simulink model "two_vector"  (R2018b)
settings: Solver=ode1  StartTime=0.0  StopTime=0.7  RelTol=1e-3
undefined symbols (not defined in the file): Ba, DiscIntNeverNeededParam, flux, Ki, Kp, L, R, states, Ts, v
libraries: powerlib x4, simulink x1
settings Model: SimulationMode=accelerator  Creator=123  LastModifiedBy=123
settings DebuggingCC: LibraryContextMissingDiagnostic=none
settings SFSimCC: SimUseLocalCustomCode=off
settings RTWCC: RTWUseLocalCustomCode=off

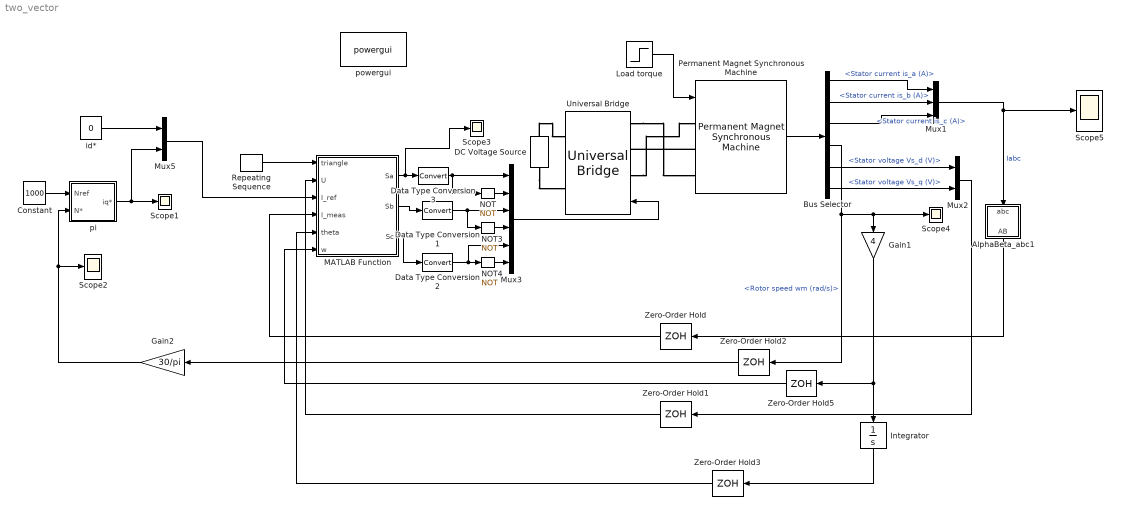
== system two_vector ==
  AlphaBeta_abc1 : Subsystem
  Bus Selector : BusSelector  OutputSignals=Stator current is_a (A),Stator current is_b (A),Stator current is_c (A),Rotor speed wm (rad/s),Stator voltage Vs_d (V),Stator voltage Vs_q (V)
  Constant : Constant  Value=1000
  DC Voltage Source : powerlib/Electrical Sources/DC Voltage Source  Amplitude=520  Measurements=None
      settings: SourceProductName=Simscape Electrical
  Data Type Conversion1 : DataTypeConversion
  Data Type Conversion2 : DataTypeConversion
  Data Type Conversion3 : DataTypeConversion
  Gain1 : Gain  Gain=4
  Gain2 : Gain  Gain=30/pi
  Integrator : Integrator
  Load torque : Step  Time=0.35  After=5  SampleTime=5e-6
  MATLAB Function : MATLAB Function  TreatAsAtomicUnit=on  SystemSampleTime=5e-6
  Mux1 : Mux  Inputs=3
  Mux2 : Mux  Inputs=2
  Mux3 : Mux  Inputs=6
  Mux5 : Mux  Inputs=2
  NOT : Logic  Operator=NOT  IconShape=distinctive  AllPortsSameDT=off  OutDataTypeStr=boolean
  NOT3 : Logic  Operator=NOT  IconShape=distinctive  AllPortsSameDT=off  OutDataTypeStr=boolean
  NOT4 : Logic  Operator=NOT  IconShape=distinctive  AllPortsSameDT=off  OutDataTypeStr=boolean
  Permanent Magnet Synchronous Machine : powerlib/Machines/Permanent Magnet Synchronous Machine  NbPhases=3  FluxDistribution=Sinusoidal  RotorType=Round  MechanicalLoad=Torque Tm  PresetModel=No  ShowDetailedParameters=on  MeasurementBus=off  Resistance=0.958  Inductance=8.5e-3  dqInductances=[5.25e-3,12e-3]  La=6e-3  MachineConstant=Flux linkage established by magnets (V.s)  Flux=0.1827  VoltageCst=132.5525  TorqueCst=1.0962  Flat=120  Mechanical=[0.003 0.008 4 0]  PolePairs=4  InitialConditions=[0,0, 0,0]  InitialConditions5ph=[0 0 0 0 0 0]  TsPowergui=0  TsBlock=1e-6  RefAngle=Aligned with phase A axis (original Park)
  Repeating Sequence : simulink/Sources/Repeating Sequence  rep_seq_t=[0 5e-6]  rep_seq_y=[0 5e-6]
  Scope{1..5} (5 alike) : Scope
  Universal Bridge : powerlib/Power Electronics/Universal Bridge  Arms=3  SnubberResistance=1e5  SnubberCapacitance=inf  Device=IGBT / Diodes  Ron=1e-3  Lon=0  ForwardVoltages="[  0  0  ]"  ForwardVoltage=0  GTOparameters=[ 10e-6 , 20e-6 ]  IGBTparameters=[ 1e-6 , 2e-6 ]  Measurements=None  Measurements_2=None  converterType=Rectifier
      settings: SourceProductName=Simscape Electrical
  Zero-Order Hold{,1..3,5} (5 alike) : ZeroOrderHold  SampleTime=5e-6
  id* : Constant  Value=0
  pi : Subsystem
  powergui : powerlib/powergui  Priority=1  SimulationMode=Discrete  SampleTime=1e-6  frequency=60  Iterations=50  frequencyindice=0  Pbase=100e6  ErrMax=1e-4  UnitsV=kV  UnitsW=MW  buscounter=0  FunctionMessages=off  echomessages=off  EnableUseOfTLC=off  CurrentSourceSwitches=off  DisableSnubberDevices=off  DisableRonSwitches=off  DisableVfSwitches=off  DisplayEquations=off  SolverType=Tustin/Backward Euler (TBE)  Interpol=off  ExternalGateDelay=off  methode=off  Ts=100  x0status=blocks  SPID=off  SwTol=0  HookPort=off  RestoreLinks=warning  ResistiveCurrentMeasurement=off  Frange=[0:2:500]  Ylog=off  Xlog=on  ShowGrid=off  save=off  variable=ZData  structure=ScopeData  ZoomFFT=off  StartTime=0.05  cycles=1  DisplayStyle=1  fundamental=50  FreqAxis=off  MaxFrequency=2000  frequencyindicesteady=1  RmsSteady=1  display=off
  wires:
  Bus Selector/3 -> Mux1/3  "<Stator current is_c (A)>"
  Mux3/1 -> Universal Bridge/1
  Data Type Conversion1/1 -> NOT3/1, Mux3/3
  Gain1/1 -> Zero-Order Hold5/1, Integrator/1
  Bus Selector/4 -> Gain1/1, Scope4/1, Zero-Order Hold2/1  "<Rotor speed wm (rad/s)>"
  NOT3/1 -> Mux3/4
  Bus Selector/2 -> Mux1/2  "<Stator current is_b (A)>"
  Permanent Magnet Synchronous Machine/1 -> Bus Selector/1
  NOT4/1 -> Mux3/6
  id*/1 -> Mux5/1
  Gain2/1 -> Scope2/1, pi/2(N*)
  Constant/1 -> pi/1(Nref)
  pi/1(iq*) -> Mux5/2, Scope1/1
  Mux1/1 -> Scope5/1, AlphaBeta_abc1/1(abc)  "Iabc"
  MATLAB Function/1(Sa) -> Data Type Conversion3/1, Scope3/1
  MATLAB Function/3(Sc) -> Data Type Conversion2/1
  Bus Selector/1 -> Mux1/1  "<Stator current is_a (A)>"
  Data Type Conversion2/1 -> Mux3/5, NOT4/1
  NOT/1 -> Mux3/2
  Repeating Sequence/1 -> MATLAB Function/1(triangle)
  Data Type Conversion3/1 -> NOT/1, Mux3/1
  AlphaBeta_abc1/1(AB) -> Zero-Order Hold/1
  Integrator/1 -> Zero-Order Hold3/1
  Bus Selector/5 -> Mux2/1  "<Stator voltage Vs_d (V)>"
  Bus Selector/6 -> Mux2/2  "<Stator voltage Vs_q (V)>"
  Mux2/1 -> Zero-Order Hold1/1
  Load torque/1 -> Permanent Magnet Synchronous Machine/1
  MATLAB Function/2(Sb) -> Data Type Conversion1/1
  Zero-Order Hold/1 -> MATLAB Function/4(I_meas)
  Zero-Order Hold1/1 -> MATLAB Function/2(U)
  Zero-Order Hold2/1 -> Gain2/1
  Zero-Order Hold3/1 -> MATLAB Function/5(theta)
  Zero-Order Hold5/1 -> MATLAB Function/6(w)
  Mux5/1 -> MATLAB Function/3(I_ref)
  connections:
  Universal Bridge/LConn1 -- Permanent Magnet Synchronous Machine/LConn1
  DC Voltage Source/RConn1 -- Universal Bridge/RConn1
  Permanent Magnet Synchronous Machine/LConn2 -- Universal Bridge/LConn2
  Universal Bridge/LConn3 -- Permanent Magnet Synchronous Machine/LConn3
  DC Voltage Source/LConn1 -- Universal Bridge/RConn2

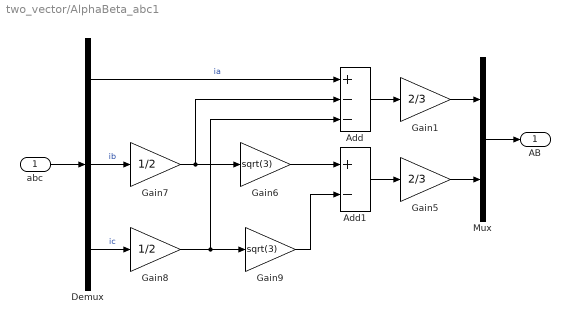
== system two_vector/AlphaBeta_abc1 ==
  abc : Inport
  Add : Sum  Inputs=+--
  Add1 : Sum  Inputs=+-
  Demux : Demux  Outputs=3
  Gain1 : Gain  Gain=2/3
  Gain5 : Gain  Gain=2/3
  Gain6 : Gain  Gain=sqrt(3)
  Gain7 : Gain  Gain=1/2
  Gain8 : Gain  Gain=1/2
  Gain9 : Gain  Gain=sqrt(3)
  Mux : Mux  Inputs=2
  AB : Outport
  wires:
  abc/1 -> Demux/1
  Demux/2 -> Gain7/1  "ib"
  Demux/3 -> Gain8/1  "ic"
  Add/1 -> Gain1/1
  Gain7/1 -> Gain6/1, Add/2
  Gain8/1 -> Gain9/1, Add/3
  Gain6/1 -> Add1/1
  Gain9/1 -> Add1/2
  Demux/1 -> Add/1  "ia"
  Add1/1 -> Gain5/1
  Gain1/1 -> Mux/1
  Gain5/1 -> Mux/2
  Mux/1 -> AB/1

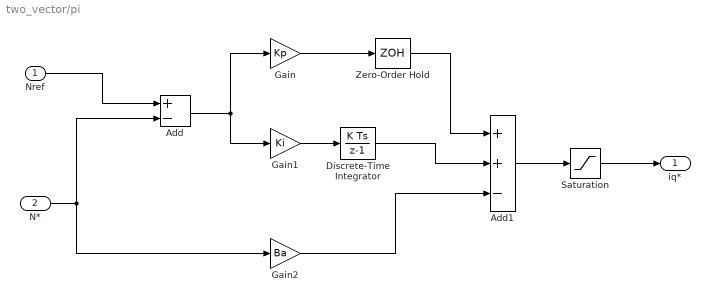
== system two_vector/pi ==
  Nref : Inport
  N* : Inport  Port=2
  Add : Sum  Inputs=+-
  Add1 : Sum  Inputs=++-
  Discrete-Time Integrator : DiscreteIntegrator  SampleTime=-1  ICPrevOutput=DiscIntNeverNeededParam  ICPrevScaledInput=DiscIntNeverNeededParam
  Gain : Gain  Gain=Kp
  Gain1 : Gain  Gain=Ki
  Gain2 : Gain  Gain=Ba
  Saturation : Saturate  UpperLimit=50  LowerLimit=-50
  Zero-Order Hold : ZeroOrderHold  SampleTime=-1
  iq* : Outport
  wires:
  Nref/1 -> Add/1
  N*/1 -> Gain2/1, Add/2
  Add/1 -> Gain1/1, Gain/1
  Gain/1 -> Zero-Order Hold/1
  Zero-Order Hold/1 -> Add1/1
  Gain1/1 -> Discrete-Time Integrator/1
  Discrete-Time Integrator/1 -> Add1/2
  Gain2/1 -> Add1/3
  Add1/1 -> Saturation/1
  Saturation/1 -> iq*/1

== matlab function two_vector/MATLAB Function ==
  data: triangle input; Sa output; U input; I_ref input; I_meas input; theta input; Sb output; Sc output; R parameter; L parameter; Ts parameter; v parameter; states parameter; w input; flux parameter

function [Sa,Sb,Sc] = control(triangle,U,I_ref,I_meas,theta, R, L, Ts, v, states,w, flux)

% persistent i_old v_last
% if isempty(v_last), v_last = 0+1j*0; end
% if isempty(i_old), i_old = 0+1j*0; end


ik_ref = (I_ref(1) + 1j*I_ref(2))*exp(1j*theta);

uk = (U(1) + 1j*U(2))*exp(1j*theta);
ik = I_meas(1) + 1j*I_meas(2);



%e = v_last - R*(ik+i_old)/2-(L/Ts)*(ik-i_old);
e = 1j*w*flux*exp(1j*theta);

% i_old = ik;
% v_last = uk;


ik1 = ik + Ts/L*(uk-R*ik-e);
us = R*ik1 + L*(ik_ref-ik1)/Ts + e;
a=mod(angle(us)+pi/6,2*pi);

n = floor(a*3/pi)+1;
if n>6
    n=1;
end

n = n + 1;
u_opt = v(n);
t_opt = Ts*real(conj(us)*u_opt)/abs(u_opt)^2;
t_opt = min((max(t_opt,0)),Ts);

% d = t_opt/Ts;
% v_last = u_opt*d;




if (triangle<=t_opt)
    Sa = states(n,1);
    Sb = states(n,2);
    Sc = states(n,3);
else
    if n==2 || n==4 || n==6
        Sa = 1;
        Sb = 1;
        Sc = 1;
    else
       Sa = 0;
       Sb = 0;
       Sc = 0;
    end
end
